simulink model "microgrid"  (R2025a)
settings: Solver=VariableStepAuto  StartTime=0.0  StopTime=10.0  RelTol=1e-3
undefined symbols (not defined in the file): Ion, Lithium, sigbuilder_block
libraries: spsMeanLib x7, spsSeriesRLCBranchLib x6, spsIGBTDiodeLib x4, spsPWMGeneratorDCDCLib x2, spsVoltageMeasurementLib x2, spsBatteryLib x1, spsCurrentMeasurementLib x1, spsDiodeLib x1, spsIGBTLib x1, spsSeriesRLCLoadLib x1, simulink x1, slpidlib x1
settings Model: Creator=ASUS  LastModifiedBy=sivas

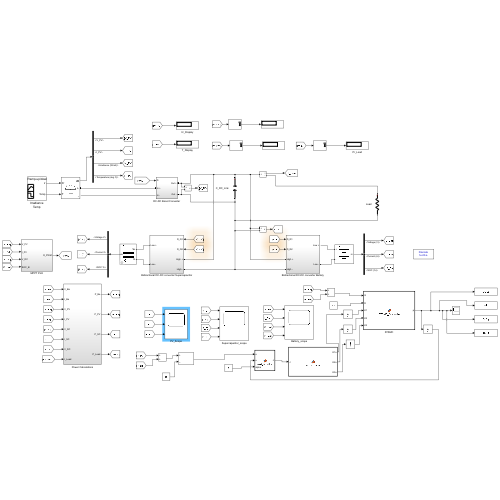
[thumbnail: Simulink's stored preview of the top-level diagram]
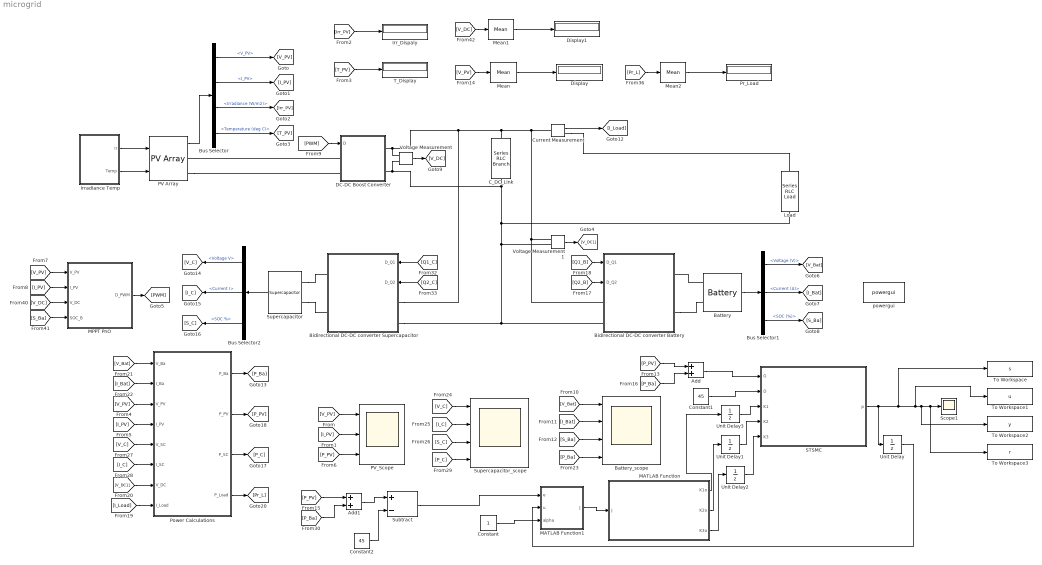
== system microgrid ==
  Add : Sum
  Add1 : Sum
  Battery : spsBatteryLib/Battery  BatType=Lithium-Ion  NomV=50  NomQ=15  SOC=100  Batt_Tr=0.1  PresetModel=on  MaxQ=15  MinV=37.5  FullV=58.1994  Dis_rate=6.5217  R=0.033333  Normal_OP=13.5652  expZone="[54.0193     0.736957]"
      settings: LibrarySourceBlock=electricdrivelib/Extra Sources/Battery
  "Battery_scope " : Scope  NumInputPorts=4
      settings: ActiveDisplayYMinimum=24.95268  ActiveDisplayYMaximum=26.67849
  Bidirectional DC-DC converter Battery : Subsystem
  Bidirectional DC-DC converter Supercapacitor : Subsystem
  Bus Selector : BusSelector  OutputSignals=V_PV,I_PV,Irradiance (W/m2),Temperature (deg C)
  Bus Selector1 : BusSelector  OutputSignals=Voltage (V),Current (A),SOC (%)
  Bus Selector2 : BusSelector  OutputSignals=Voltage V,Current I,SOC %
  C_DC_Link : spsSeriesRLCBranchLib/Series RLC Branch  LConnTagsString=__new0  RConnTagsString=__new0  BranchType=C  Resistance=1  Inductance=1e-3  SetiL0=off  InitialCurrent=0  Capacitance=300e-6  Setx0=off  InitialVoltage=0  Measurements=None
  Constant : Constant
  Constant1 : Constant  Value=45
  Constant2 : Constant  Value=45
  Current Measurement : spsCurrentMeasurementLib/Current Measurement  PhasorSimulation=off  OutputType=Complex  PSBequivalent=0
  DC-DC Boost Converter : Subsystem
  Display : Display
  Display1 : Display
  Irr_Dispaly : Display
  Irradiance Temp : Subsystem  Tag=STV Subsys  LoadFcn=sigbuilder_block('load');  StartFcn=sigbuilder_block('start');  StopFcn=sigbuilder_block('stop');  ClipboardFcn=sigbuilder_block('clipboard');  mask(Sigbuilder block){tuvar=[0:10]}
      mask help: Sigbuilder GUI
      mask init:
      | if ~strcmp(get_param(bdroot(gcbh),'SimulationStatus'),'stopped') tuvar = sigbuilder_block('maskInit'); end
      settings: CopyFcn=sigbuilder_block('copy');  DeleteFcn=sigbuilder_block('delete');  ModelCloseFcn=sigbuilder_block('modelClose');  PreSaveFcn=sigbuilder_block('preSave');  PauseFcn=sigbuilder_block('pause')  ContinueFcn=sigbuilder_block('continue')  NameChangeFcn=sigbuilder_block('namechange');  OpenFcn=sigbuilder_block('open',[316.5 171.75 805.5 485.25 ]);  CloseFcn=sigbuilder_block('close');
      mask Display: plot(0, 0, 100, 100,[2, 2, 32, 32, 2], [68, 8, 8, 68, 68],[32, 2], [38, 38], [32, 19, 2],[53, 60, 44], [32, 17, 17, 2],[16, 16, 31, 31]);txt = getActiveGroup(gcbh);text(2, 100, txt,'verticalAlignment', 'top');
  Load : spsSeriesRLCLoadLib/Series RLC Load  LConnTagsString=a  RConnTagsString=__new0  NominalVoltage=50  NominalFrequency=0.00001  ActivePower=500  InductivePower=0  CapacitivePower=0  Setx0=off  InitialVoltage=0  SetiL0=off  InitialCurrent=0  Measurements=None  LoadType=constant Z
  MATLAB Function : MATLAB Function  TreatAsAtomicUnit=on
  MATLAB Function1 : MATLAB Function  TreatAsAtomicUnit=on
  MPPT PnO : Subsystem
  Mean : spsMeanLib/Mean  Freq=50  Vinit=0  Ts=0
  Mean1 : spsMeanLib/Mean  Freq=50  Vinit=0  Ts=0
  Mean2 : spsMeanLib/Mean  Freq=60  Vinit=0  Ts=0
  PV Array : spsPVArrayLib/PV Array  Npar=4  Nser=2  PlotType=one module @ 25 deg.C & specified irradiances  S_vec="[ 1000 800 500  250 ]"  Temp_C_vec="[0 25 50  ]"  ModuleName=Waaree Energies WU-120  PlotWhenSelected=on  Pm=120.7  Ncell=72  Voc=21  Isc=8  Vm=17  Im=7.1  beta_Voc_pc=-0.358  alpha_Isc_pc=0.052  beta_Voc=-0.07518  alpha_Isc=0.00416  IL=8.0502  I0=2.411e-10  nI=0.47063  Rsh=31.6819  Rs=0.19891  RobustModel=off  RobustCellTemperature=313.3991  BAL=on  Tc=Tc  Tfilter=5e-5
  PV_Scope : Scope  NumInputPorts=3
      settings: ActiveDisplayYMinimum=-7.4542805917151895  ActiveDisplayYMaximum=46.05818124761776  DataLoggingVariableName=ScopeData2
  Power Calculations : Subsystem
  Pr_Load : Display
  STSMC : MATLAB Function  TreatAsAtomicUnit=on
  Scope1 : Scope
      settings: ActiveDisplayYMinimum=-26.055849756366086  ActiveDisplayYMaximum=-15.511026218446876  DataLoggingVariableName=ScopeData4
  Subtract : Sum  Inputs=+-
  Supercapacitor : spsSupercapacitorLib/Supercapacitor  C=29  Rdc=0.003  Voltage=32  Ns=1  Np=1  Vinit=32  Temp=25  Nc=1  r=1e-9  epsilon=6.0208e-10  Ioc=10  Vself="[48  47.8  47.06  44.65]"
      settings: LibrarySourceBlock=electricdrivelib/Extra Sources/Supercapacitor
  Supercapacitor_scope : Scope  NumInputPorts=4
      settings: ActiveDisplayYMinimum=31.982834502483911  ActiveDisplayYMaximum=32.00186521718993
  T_Display : Display
  To Workspace : ToWorkspace  VariableName=s  SampleTime=-1
  To Workspace1 : ToWorkspace  VariableName=u  SampleTime=-1
  To Workspace2 : ToWorkspace  VariableName=y  SampleTime=-1
  To Workspace3 : ToWorkspace  VariableName=r  SampleTime=-1
  Unit Delay{,1..3} (4 alike) : UnitDelay  InitialCondition=1  SampleTime=-1  HasFrameUpgradeWarning=on
  Voltage Measurement : spsVoltageMeasurementLib/Voltage Measurement  PhasorSimulation=off  OutputType=Complex  PSBequivalent=0
  Voltage Measurement1 : spsVoltageMeasurementLib/Voltage Measurement  PhasorSimulation=off  OutputType=Complex  PSBequivalent=0
  powergui : spspowerguiLib/powergui  Priority=1  SimulationMode=Discrete  SampleTime=1e-6  frequency=60  Iterations=50  frequencyindice=0  Pbase=100e6  ErrMax=1e-4  UnitsV=kV  UnitsW=MW  buscounter=0  FunctionMessages=off  echomessages=off  EnableUseOfTLC=off  CurrentSourceSwitches=off  DisableSnubberDevices=off  DisableRonSwitches=off  DisableVfSwitches=off  DisplayEquations=off  AutomaticDiscreteSolvers=off  SolverType=Tustin/Backward Euler (TBE)  Interpol=off  ExternalGateDelay=off  methode=off  Ts=100  x0status=blocks  SPID=on  SwTol=0  HookPort=off  NonlinearTolerance=1e-4  nMaxIteration=100  ContinueOnMaxIteration=off  RestoreLinks=warning  ResistiveCurrentMeasurement=off  Frange=[0:2:500]  Ylog=off  Xlog=on  ShowGrid=off  save=off  variable=ZData  structure=0  ZoomFFT=off  StartTime=0.0  cycles=1  DisplayStyle=1  fundamental=60  FreqAxis=off  MaxFrequency=1000  frequencyindicesteady=1  RmsSteady=1  display=off
  wires:
  Irradiance Temp/2(Temp) -> PV Array/2
  Current Measurement/1 -> [I_Load]
  Bus Selector1/3 -> [S_Ba]  "<SOC (%)>"
  Bus Selector/3 -> [Irr_PV]  "<Irradiance (W/m2)>"
  [S_Ba] -> MPPT PnO/4(SOC_B)
  PV Array/1 -> Bus Selector/1
  [Q1_B] -> Bidirectional DC-DC converter Battery/1(D_Q1)
  [Q1_C] -> Bidirectional DC-DC converter Supercapacitor/1(D_Q1)
  Mean/1 -> Display/1
  [V_DC] -> Mean1/1
  Irradiance Temp/1(Ir) -> PV Array/1
  Supercapacitor/1 -> Bus Selector2/1
  [V_DC] -> MPPT PnO/3(V_DC)
  [Q2_B] -> Bidirectional DC-DC converter Battery/2(D_Q2)
  [Pr_L] -> Mean2/1
  [Q2_C] -> Bidirectional DC-DC converter Supercapacitor/2(D_Q2)
  Bus Selector1/1 -> [V_Bat]  "<Voltage (V)>"
  MPPT PnO/1(D_PWM) -> [PWM]
  [V_PV] -> MPPT PnO/1(V_PV)
  Bus Selector2/2 -> [I_C]  "<Current I>"
  Bus Selector1/2 -> [I_Bat]  "<Current (A)>"
  [PWM] -> DC-DC Boost Converter/1(D)
  Mean1/1 -> Display1/1
  Bus Selector2/1 -> [V_C]  "<Voltage V>"
  Mean2/1 -> Pr_Load/1
  [I_PV] -> MPPT PnO/2(I_PV)
  Bus Selector2/3 -> [S_C]  "<SOC %>"
  Bus Selector/4 -> [T_PV]  "<Temperature (deg C)>"
  Voltage Measurement/1 -> [V_DC]
  [Irr_PV] -> Irr_Dispaly/1
  Bus Selector/2 -> [I_PV]  "<I_PV>"
  Bus Selector/1 -> [V_PV]  "<V_PV>"
  [T_PV] -> T_Display/1
  [V_PV] -> Mean/1
  Battery/1 -> Bus Selector1/1
  [I_Load] -> Power Calculations/8(I_Load)
  Power Calculations/2(P_PV) -> [P_PV]
  [V_Bat] -> Power Calculations/1(V_Ba)
  Power Calculations/4(P_Load) -> [Pr_L]
  [V_C] -> Power Calculations/5(V_SC)
  [V_PV] -> Power Calculations/3(V_PV)
  Power Calculations/3(P_SC) -> [P_C]
  Power Calculations/1(P_Ba) -> [P_Ba]
  [I_PV] -> Power Calculations/4(I_PV)
  [V_DC1] -> Power Calculations/7(V_DC)
  [I_C] -> Power Calculations/6(I_SC)
  [I_Bat] -> Power Calculations/2(I_Ba)
  [I_Bat] -> "Battery_scope "/2
  [V_Bat] -> "Battery_scope "/1
  [S_C] -> Supercapacitor_scope/3
  [V_PV] -> PV_Scope/1
  [I_C] -> Supercapacitor_scope/2
  [S_Ba] -> "Battery_scope "/3
  [I_PV] -> PV_Scope/2
  [P_Ba] -> "Battery_scope "/4
  [P_PV] -> PV_Scope/3
  [V_C] -> Supercapacitor_scope/1
  [P_C] -> Supercapacitor_scope/4
  Voltage Measurement1/1 -> [V_DC1]
  Subtract/1 -> MATLAB Function1/1(e)
  STSMC/1(p) -> Unit Delay/1, To Workspace/1, To Workspace1/1, To Workspace2/1, Scope1/1, To Workspace3/1
  Constant/1 -> MATLAB Function1/3(alpha)
  MATLAB Function1/1(J) -> MATLAB Function/1(J)
  Constant1/1 -> STSMC/2(D)
  Unit Delay/1 -> MATLAB Function1/2(u)
  MATLAB Function/1(K1o) -> Unit Delay3/1
  MATLAB Function/2(K2o) -> Unit Delay1/1
  MATLAB Function/3(K3o) -> Unit Delay2/1
  Unit Delay2/1 -> STSMC/5(K3)
  Unit Delay1/1 -> STSMC/4(K2)
  Unit Delay3/1 -> STSMC/3(K1)
  [P_PV] -> Add/1
  [P_Ba] -> Add/2
  Add/1 -> STSMC/1(G)
  [P_PV] -> Add1/1
  [P_Ba] -> Add1/2
  Add1/1 -> Subtract/1
  Constant2/1 -> Subtract/2
  connections:
  Bidirectional DC-DC converter Battery/LConn2 -- Voltage Measurement1/LConn2 -- Voltage Measurement/LConn2 -- DC-DC Boost Converter/RConn2 -- C_DC_Link/RConn1 -- Load/RConn1 -- Bidirectional DC-DC converter Supercapacitor/LConn2
  DC-DC Boost Converter/RConn1 -- Voltage Measurement1/LConn1 -- Bidirectional DC-DC converter Battery/LConn1 -- Current Measurement/LConn1 -- C_DC_Link/LConn1 -- Bidirectional DC-DC converter Supercapacitor/LConn1 -- Voltage Measurement/LConn1
  DC-DC Boost Converter/LConn1 -- PV Array/RConn1
  Supercapacitor/LConn2 -- Bidirectional DC-DC converter Supercapacitor/RConn2
  Bidirectional DC-DC converter Battery/RConn2 -- Battery/LConn2
  PV Array/RConn2 -- DC-DC Boost Converter/LConn2
  Battery/LConn1 -- Bidirectional DC-DC converter Battery/RConn1
  Current Measurement/RConn1 -- Load/LConn1
  Supercapacitor/LConn1 -- Bidirectional DC-DC converter Supercapacitor/RConn1

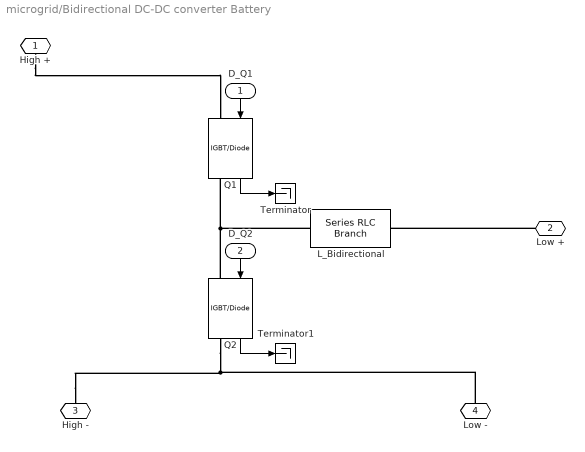
== system microgrid/Bidirectional DC-DC converter Battery ==
  D_Q1 : Inport
  D_Q2 : Inport  Port=2
  L_Bidirectional : spsSeriesRLCBranchLib/Series RLC Branch  LConnTagsString=__new0  RConnTagsString=__new0  BranchType=RL  Resistance=0.05  Inductance=0.3e-3  SetiL0=off  InitialCurrent=0  Capacitance=1e-6  Setx0=off  InitialVoltage=0  Measurements=None
  Q1 : spsIGBTDiodeLib/IGBT//Diode  Ron=1e-3  Rs=1e5  Cs=inf  Measurements=on
  Q2 : spsIGBTDiodeLib/IGBT//Diode  Ron=1e-3  Rs=1e5  Cs=inf  Measurements=on
  Terminator : Terminator
  Terminator1 : Terminator
  High + : PMIOPort  Side=Left
  Low + : PMIOPort  Port=2  Side=Right
  High - : PMIOPort  Port=3  Side=Left
  Low - : PMIOPort  Port=4  Side=Right
  wires:
  D_Q2/1 -> Q2/1
  D_Q1/1 -> Q1/1
  Q1/1 -> Terminator/1
  Q2/1 -> Terminator1/1
  connections:
  High -/RConn1 -- Low -/RConn1 -- Q2/RConn1
  High +/RConn1 -- Q1/LConn1
  Low +/RConn1 -- L_Bidirectional/RConn1
  Q2/LConn1 -- L_Bidirectional/LConn1 -- Q1/RConn1

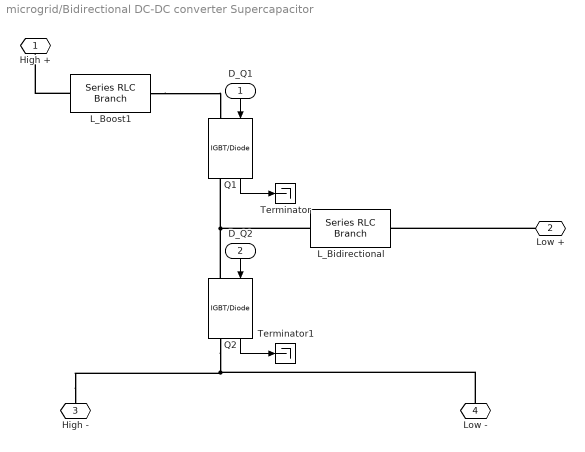
== system microgrid/Bidirectional DC-DC converter Supercapacitor ==
  D_Q1 : Inport
  D_Q2 : Inport  Port=2
  L_Bidirectional : spsSeriesRLCBranchLib/Series RLC Branch  LConnTagsString=__new0  RConnTagsString=__new0  BranchType=RL  Resistance=0.05  Inductance=0.355e-3  SetiL0=off  InitialCurrent=0  Capacitance=1e-6  Setx0=off  InitialVoltage=0  Measurements=None
  L_Boost1 : spsSeriesRLCBranchLib/Series RLC Branch  LConnTagsString=__new0  RConnTagsString=__new0  BranchType=L  Resistance=0.05  Inductance=1.5e-3  SetiL0=off  InitialCurrent=0  Capacitance=1e-6  Setx0=off  InitialVoltage=0  Measurements=None
  Q1 : spsIGBTDiodeLib/IGBT//Diode  Ron=1e-3  Rs=1e5  Cs=inf  Measurements=on
  Q2 : spsIGBTDiodeLib/IGBT//Diode  Ron=1e-3  Rs=1e5  Cs=inf  Measurements=on
  Terminator : Terminator
  Terminator1 : Terminator
  High + : PMIOPort  Side=Left
  Low + : PMIOPort  Port=2  Side=Right
  High - : PMIOPort  Port=3  Side=Left
  Low - : PMIOPort  Port=4  Side=Right
  wires:
  D_Q2/1 -> Q2/1
  D_Q1/1 -> Q1/1
  Q1/1 -> Terminator/1
  Q2/1 -> Terminator1/1
  connections:
  High -/RConn1 -- Low -/RConn1 -- Q2/RConn1
  Low +/RConn1 -- L_Bidirectional/RConn1
  Q2/LConn1 -- L_Bidirectional/LConn1 -- Q1/RConn1
  L_Boost1/RConn1 -- Q1/LConn1
  L_Boost1/LConn1 -- High +/RConn1

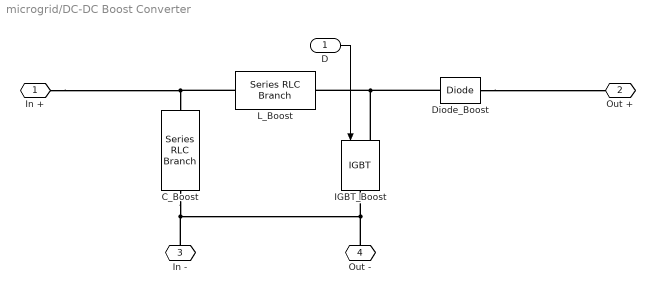
== system microgrid/DC-DC Boost Converter ==
  D : Inport
  C_Boost : spsSeriesRLCBranchLib/Series RLC Branch  LConnTagsString=__new0  RConnTagsString=__new0  BranchType=C  Resistance=0.01  Inductance=1e-3  SetiL0=off  InitialCurrent=0  Capacitance=2200e-6  Setx0=off  InitialVoltage=0  Measurements=None
  Diode_Boost : spsDiodeLib/Diode  Ron=1e-4  Lon=0  Vf=0  IC=0  UseSnubber=off  Rs=inf  Cs=inf  Measurements=off
  IGBT_Boost : spsIGBTLib/IGBT  Ron=0.001  Lon=0  Vf=0  Tf=0  Tt=0  IC=0  Rs=1e5  Cs=inf  Measurements=off
  L_Boost : spsSeriesRLCBranchLib/Series RLC Branch  LConnTagsString=__new0  RConnTagsString=__new0  BranchType=RL  Resistance=0.05  Inductance=0.352e-3  SetiL0=off  InitialCurrent=0  Capacitance=1e-6  Setx0=off  InitialVoltage=0  Measurements=None
  In + : PMIOPort  Side=Left
  Out + : PMIOPort  Port=2  Side=Right
  In - : PMIOPort  Port=3  Side=Left
  Out - : PMIOPort  Port=4  Side=Right
  wires:
  D/1 -> IGBT_Boost/1
  connections:
  IGBT_Boost/LConn1 -- Diode_Boost/LConn1 -- L_Boost/RConn1
  Diode_Boost/RConn1 -- Out +/RConn1
  L_Boost/LConn1 -- In +/RConn1 -- C_Boost/LConn1
  C_Boost/RConn1 -- In -/RConn1 -- Out -/RConn1 -- IGBT_Boost/RConn1

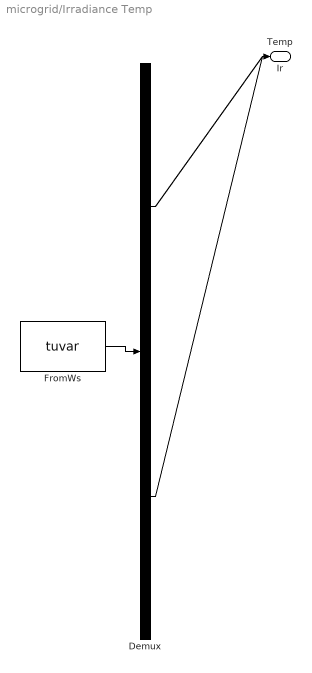
== system microgrid/Irradiance Temp ==
  Demux : Demux  Tag=STV Demux  Outputs=2
      settings: DisplayOption=none
  FromWs : FromWorkspace  Tag=STV FromWs  VariableName=tuvar
      SigBuilderData=|
      | common.afterFinalStr = 'Extrapolate'
      | common.sampleTime = '0'
      | dataSet(1).timeRange = [0 2]
      | dataSet(1).name = 'Constant Irradiance'
      | dataSet(2).timeRange = [0 4]
      | dataSet(2).name = 'Step Irradiance'
      | dataSet(3).timeRange = [0 2]
      | dataSet(3).name = 'Ramp-up/down Irradiance'
      | sbobj.Groups(1).Name = 'Constant Irradiance'
      | sbobj.Groups(1).Signals(1).Name = 'Ir'
      | sbobj.Groups(1).Signals(1).XData = [0 2]
      | sbobj.Groups(1).Signals(1).YData = [1000 1000]
      | sbobj.Groups(1).Signals(2).Name = 'Temp'
      | sbobj.Groups(1).Signals(2).XData = [0 1 1 2]
      | sbobj.Groups(1).Signals(2).YData = [0 0 1 1]
      | sbobj.Groups(1).TimeRange = [0 2]
      | sbobj.Groups(2).Name = 'Step Irradiance'
      | sbobj.Groups(2).Signals(1).Name = 'Ir'
      | sbobj.Groups(2).Signals(1).XData = [0 1 1 4]
      | sbobj.Groups(2).Signals(1).YData = [1000 1000 800 800]
      | sbobj.Groups(2).Signals(2).Name = 'Temp'
      | sbobj.Groups(2).Signals(2).XData = [0 1 1 4]
      | sbobj.Groups(2).Signals(2).YData = [0 0 1 1]
      | sbobj.Groups(2).TimeRange = [0 4]
      | sbobj.Groups(3).Name = 'Ramp-up/down Irradiance'
      | sbobj.Groups(3).Signals(1).Name = 'Ir'
      | sbobj.Groups(3).Signals(1).XData = [0 0.985 0.985 2]
      | sbobj.Groups(3).Signals(1).YData = [980 665 645 465]
      | sbobj.Groups(3).Signals(2).Name = 'Temp'
      | sbobj.Groups(3).Signals(2).XData = [0 2]
      | sbobj.Groups(3).Signals(2).YData = [25 25]
      | sbobj.Groups(3).TimeRange = [0 2]
  Ir : Outport  Tag=STV Outport
  Temp : Outport  Tag=STV Outport  Port=2
  wires:
  FromWs/1 -> Demux/1
  Demux/1 -> Ir/1
  Demux/2 -> Temp/1

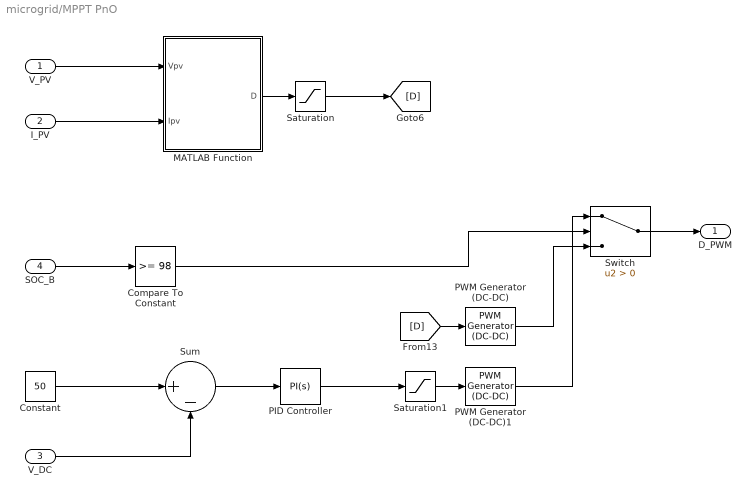
== system microgrid/MPPT PnO ==
  V_PV : Inport
  I_PV : Inport  Port=2
  V_DC : Inport  Port=3
  SOC_B : Inport  Port=4
  Compare To Constant : simulink/Logic and Bit Operations/Compare To Constant  relop=>=  const=98  OutDataTypeStr=boolean
  Constant : Constant  Value=50
  MATLAB Function : MATLAB Function  TreatAsAtomicUnit=on
  PID Controller : slpidlib/PID Controller  Controller=PI  Form=Parallel  TimeDomain=Continuous-time  UseExternalTs=off  SampleTime=-1  IntegratorMethod=Forward Euler  FilterMethod=Forward Euler  ControllerParametersSource=internal  P=0.1  I=0.1  UseKiTs=off  D=0  UseExternalDerivativeSource=off  N=100  UseFilter=on  TunerSelectOption=Transfer Function Based (PID Tuner App)  InitialConditionSource=internal  InitialConditionForIntegrator=0  InitialConditionForFilter=0  DifferentiatorICPrevScaledInput=0  ExternalReset=none  TrackingMode=off  Kt=1  LimitOutput=off  SatLimitsSource=internal  UpperSaturationLimit=inf  LowerSaturationLimit=-inf  LinearizeAsGain=on  AntiWindupMode=none  Kb=1  LimitIntegrator=off  UpperIntegratorSaturationLimit=inf  LowerIntegratorSaturationLimit=-inf  POutMin=[]  POutMax=[]  IOutMin=[]  IOutMax=[]  DOutMin=[]  DOutMax=[]  NOutMin=[]  NOutMax=[]  SumOutMin=[]  SumOutMax=[]  SaturationOutMin=[]  SaturationOutMax=[]  PParamMin=[]  PParamMax=[]  IParamMin=[]  IParamMax=[]  DParamMin=[]  DParamMax=[]  NParamMin=[]  NParamMax=[]  KbParamMin=[]  KbParamMax=[]  KtParamMin=[]  KtParamMax=[]  KbOutMin=[]  KbOutMax=[]  KtOutMin=[]  KtOutMax=[]  IntegratorOutMin=[]  IntegratorOutMax=[]  FilterOutMin=[]  FilterOutMax=[]  SumI1OutMin=[]  SumI1OutMax=[]  SumI2OutMin=[]  SumI2OutMax=[]  SumI3OutMin=[]  SumI3OutMax=[]  SumI4OutMin=[]  SumI4OutMax=[]  SumDOutMin=[]  SumDOutMax=[]  DifferentiatorOutMin=[]  DifferentiatorOutMax=[]  FilterDiffOutCoefMin=[]  FilterDiffOutCoefMax=[]  ReciprocalOutMin=[]  ReciprocalOutMax=[]  SumDenOutMin=[]  SumDenOutMax=[]  SumNumOutMin=[]  SumNumOutMax=[]  DivideOutMin=[]  DivideOutMax=[]  UdiffTsProdOutMin=[]  UdiffTsProdOutMax=[]  NTsProdOutMin=[]  NTsProdOutMax=[]  UintegralTsProdOutMin=[]  UintegralTsProdOutMax=[]  UngainTsProdOutMin=[]  UngainTsProdOutMax=[]  ClampingZeroOutDataTypeStr=Inherit: Inherit via back propagation  ClampingZeroOutMin=[]  ClampingZeroOutMax=[]  FilterDenConstantOutDataTypeStr=Inherit: Inherit via back propagation  FilterDenConstantOutMin=[]  FilterDenConstantOutMax=[]  PCopyOutDataTypeStr=Inherit: Inherit via back propagation  PCopyOutMin=[]  PCopyOutMax=[]  NCopyOutDataTypeStr=Inherit: Inherit via back propagation  NCopyOutMin=[]  NCopyOutMax=[]  IntegratorContinuousStateAttributes=''  IntegratorStateMustResolveToSignalObject=off  IntegratorRTWStateStorageClass=Auto  FilterContinuousStateAttributes=''  FilterStateMustResolveToSignalObject=off  FilterRTWStateStorageClass=Auto  ParallelPVariant=InternalParameters  IdealPVariant=Disabled  IVariant=InternalParameters  DVariant=Disabled  IntegratorVariant=Continuous  SatVariant=Disabled  AWVariant=Passthrough  PCopyVariant=Disabled  TRVariant=Disabled  FdbkBlocksVariant=Forward  IdealPFdbkVariant=Disabled  SatFdbkVariant=Disabled  DerivativeFilterVariant=Disabled  NVariant=Disabled  NCopyVariant=Disabled_SignalSpec  FilterICVariant=Disabled  IntegratorICVariant=InternalICs  ExternalResetVariant=Disabled  TRSumVariant=Passthrough  SumFdbkVariant=Disabled  SumVariant=Sum_PI  TsampFilterVariant=InternalTs  TsampNgainVariant=Passthrough  TsampIntegralVariant=Disabled_SignalSpec  ExternalSaturationOutDataTypeStr=Inherit: Same as second input  DerivativeSourceVariant=Disabled  PreIntVariant=InternalPreInt
  PWM Generator (DC-DC) : spsPWMGeneratorDCDCLib/PWM Generator (DC-DC)  Fsw=5000  Ts=0
  PWM Generator (DC-DC)1 : spsPWMGeneratorDCDCLib/PWM Generator (DC-DC)  Fsw=5000  Ts=0
  Saturation : Saturate
  Saturation1 : Saturate
  Sum : Sum  Inputs=|+-
  Switch : Switch  Criteria=u2 > Threshold  SaturateOnIntegerOverflow=off  InputSameDT=off
  D_PWM : Outport
  wires:
  Saturation/1 -> [D]
  [D] -> PWM Generator (DC-DC)/1
  I_PV/1 -> MATLAB Function/2(Ipv)
  V_PV/1 -> MATLAB Function/1(Vpv)
  MATLAB Function/1(D) -> Saturation/1
  Sum/1 -> PID Controller/1
  V_DC/1 -> Sum/2
  Constant/1 -> Sum/1
  PID Controller/1 -> Saturation1/1
  Switch/1 -> D_PWM/1
  Saturation1/1 -> PWM Generator (DC-DC)1/1
  Compare To Constant/1 -> Switch/2
  SOC_B/1 -> Compare To Constant/1
  PWM Generator (DC-DC)/1 -> Switch/3
  PWM Generator (DC-DC)1/1 -> Switch/1

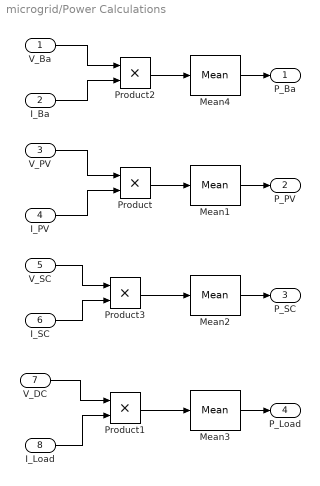
== system microgrid/Power Calculations ==
  V_Ba : Inport
  I_Ba : Inport  Port=2
  V_PV : Inport  Port=3
  I_PV : Inport  Port=4
  V_SC : Inport  Port=5
  I_SC : Inport  Port=6
  V_DC : Inport  Port=7
  I_Load : Inport  Port=8
  Mean{1..4} (4 alike) : spsMeanLib/Mean  Freq=60  Vinit=0  Ts=0
  Product{,1..3} (4 alike) : Product
  P_Ba : Outport
  P_PV : Outport  Port=2
  P_SC : Outport  Port=3
  P_Load : Outport  Port=4
  wires:
  I_Ba/1 -> Product2/2
  V_Ba/1 -> Product2/1
  V_PV/1 -> Product/1
  I_PV/1 -> Product/2
  V_DC/1 -> Product1/1
  I_Load/1 -> Product1/2
  V_SC/1 -> Product3/1
  I_SC/1 -> Product3/2
  Mean4/1 -> P_Ba/1
  Product2/1 -> Mean4/1
  Mean1/1 -> P_PV/1
  Product/1 -> Mean1/1
  Mean2/1 -> P_SC/1
  Product3/1 -> Mean2/1
  Mean3/1 -> P_Load/1
  Product1/1 -> Mean3/1

== matlab function microgrid/STSMC ==
  data: G input; p output; D input; K1 input; K2 input; K3 input
function p = STSMC_Controller(G, D, K1, K2, K3)
%#codegen
e = G - D;

% super-twisting style term |e|^(1/2)*sign(e)
st = sqrt(abs(e)) * sign(e);

p = K1*e + K2*st + K3*sign(e);
end

== matlab function microgrid/MPPT PnO/MATLAB Function ==
  settings: updateMethod=DISCRETE  sampleTime=1e-4
  data: Vpv input; D output; Ipv input
function D = PandO(Vpv,Ipv)

persistent Dold Pold Vold


if isempty(Dold)
    Dold = 0.35;
    Vold = 17;
    Pold = 120;
end


deltaD = 0.001;

Ppv = Vpv*Ipv;

if (Ppv-Pold) ~= 0
    if (Ppv-Pold) > 0
        if (Vpv-Vold) > 0
            D = Dold - deltaD;
        else
            D = Dold + deltaD;
        end
    else
        if (Vpv-Vold) > 0
            D = Dold + deltaD;
        else
            D = Dold - deltaD;
        end        
    end
else
    D = Dold;
end

Dold = D;
Vold = Vpv;
Pold = Ppv;

== matlab function microgrid/MATLAB Function ==
  data: J input; K1o output; K2o output; K3o output
function [K1o, K2o, K3o] = ACO_Tuner(J)
%#codegen
% Runs once per tuning interval. Keeps internal state across calls.
% Bounds (negative for price-demand inverse effect)
K1_min = -5;  K1_max = -0.05;
K3_min = -5;  K3_max = -0.05;
K2_min =  0;  K2_max =  1;

nAnts   = 16;        % ants per call (lightweight online ACO)
alpha   = 1.0;       % pheromone influence
beta    = 1.0;       % heuristic influence
rho     = 0.6;       % evaporation
q_ph    = 1.0;       % deposit scaling
sigmaK  = 0.35;      % exploration noise (fraction of range)

% --- persistent state across calls
persistent tau_K1 tau_K3 bestK1 bestK3 bestJ init
if isempty(init)
    tau_K1 = 1.0; tau_K3 = 1.0;     % global pheromones (scalar form)
    bestK1 = -1.0; bestK3 = -0.5;   % reasonable starting point
    bestJ  = inf;
    init = true;
end

% ---- Heuristic (use last performance as hint): prefer stronger action if J high
% simple heuristic factors (bounded 0.5..2)
hK1 = bound(0.5 + 1.5*normalize(J, 0, 1), 0.5, 2.0);
hK3 = hK1;

% --- Sample ants (roulette using tau^alpha * eta^beta)
cands = zeros(nAnts,2);
scores = zeros(nAnts,1);

for k = 1:nAnts
    % stochastic sampling around current best using pheromone/heuristic
    r1 = (rand()*2-1)*sigmaK; r3 = (rand()*2-1)*sigmaK;
    K1 = bestK1 + r1*(K1_max-K1_min);
    K3 = bestK3 + r3*(K3_max-K3_min);

    % clamp to bounds
    K1 = bound(K1, K1_min, K1_max);
    K3 = bound(K3, K3_min, K3_max);

    % score based on current observed J with mild regularization
    % (in a full co-sim you'd run a short probe; online we use latest J)
    cost = J + 0.002*(K1^2 + K3^2); 

    cands(k,:) = [K1, K3];
    scores(k)  = cost;
end

% pick best this iteration
[Ji, idx] = min(scores); 
K1b = cands(idx,1); 
K3b = cands(idx,2);

% pheromone update
tau_K1 = (1-rho)*tau_K1 + q_ph/(Ji+1e-6);
tau_K3 = (1-rho)*tau_K3 + q_ph/(Ji+1e-6);

% keep global best
if Ji < bestJ
    bestJ  = Ji; 
    bestK1 = K1b; 
    bestK3 = K3b;
end

% outputs to controller (you can low-pass them if you want)
K1o = bestK1;
K3o = bestK3;
K2o = 0.25;  % fixed; or make it a tuned variable similarly

end

% --- helpers
function y = bound(x, lo, hi)
y = min(max(x,lo),hi);
end

function y = normalize(x, lo, hi)
% maps x to ~[0,1] using rough scale (tune lo/hi to your plant)
if nargin < 2, lo = 0; end
if nargin < 3, hi = 1; end
y = (x - lo) / max(hi-lo, 1e-6);
y = min(max(y,0),1);
end

== matlab function microgrid/MATLAB Function1 ==
  settings: updateMethod=DISCRETE
  data: e input; u input; J output; alpha input
function J = cost_function(e, u, alpha)
%#codegen
persistent J_accum
if isempty(J_accum)
    J_accum = 0;
end

% Sampling time (you can set this according to your model, e.g., 0.01s)
Ts = 0.01;  

% Incremental cost
dJ = (e^2 + alpha * (u^2)) * Ts;

% Accumulate cost
J_accum = J_accum + dJ;

% Output
J = J_accum;
end
